simulink model "ROPOD_Control_incFlock_UDPTest"  (R2017b)
settings: Solver=ode1  StartTime=0.0  StopTime=Tfinal  FixedStep=Ts  RelTol=1e-3  EnableMultiTasking=on
PreLoadFcn:
  | init_model
InitFcn:
  | init_model
values from neighbouring files (symbols this model uses):
  AgentNumber = 1    [init_model.m]
  FFtheta_intia = 0    [init_model.m]
  FFxy_mass = 0*80    (= 0)    [init_model.m]
  I_fhz_ddelta_cntr = 0    [init_model.m]
  I_fhz_dtheta_cntr = 0.3    [init_model.m]
  I_fhz_dtheta_flock_cntr = 0.1    [init_model.m]
  I_fhz_dvarphi_cntr = 0    [init_model.m]
  I_fhz_dxdy_cntr = 0.25    [init_model.m]
  I_fhz_dxdy_flock_cntr = 0.1    [init_model.m]
  K_gain_ddelta_cntr = 0.1    [init_model.m]
  K_gain_dtheta_cntr = 150    [init_model.m]
  K_gain_dtheta_flock_cntr = 100    [init_model.m]
  K_gain_dvarphi_cntr = 0.05    [init_model.m]
  K_gain_dxdy_cntr = 200    [init_model.m]
  K_gain_dxdy_flock_cntr = 200    [init_model.m]
  LL_wp_fhz_ddelta_cntr = 2    [init_model.m]
  LL_wp_fhz_dtheta_cntr = 20    [init_model.m]
  LL_wp_fhz_dtheta_flock_cntr = 20    [init_model.m]
  LL_wp_fhz_dvarphi_cntr = 10    [init_model.m]
  LL_wp_fhz_dxdy_cntr = 20    [init_model.m]
  LL_wp_fhz_dxdy_flock_cntr = 20    [init_model.m]
  LL_wz_fhz_ddelta_cntr = 2    [init_model.m]
  LL_wz_fhz_dtheta_cntr = 20    [init_model.m]
  LL_wz_fhz_dtheta_flock_cntr = 20    [init_model.m]
  LL_wz_fhz_dvarphi_cntr = 2    [init_model.m]
  LL_wz_fhz_dxdy_cntr = 20    [init_model.m]
  LL_wz_fhz_dxdy_flock_cntr = 20    [init_model.m]
  LPF_fhz_ddelta_cntr = 50    [init_model.m]
  LPF_fhz_ddelta_meas = 50    [init_model.m]
  LPF_fhz_dtheta_cntr = 100    [init_model.m]
  LPF_fhz_dtheta_flock_cntr = 40    [init_model.m]
  LPF_fhz_dvarphi_cntr = 50    [init_model.m]
  LPF_fhz_dvarphi_meas = 50    [init_model.m]
  LPF_fhz_dxdy_cntr = 100    [init_model.m]
  LPF_fhz_dxdy_flock_cntr = 40    [init_model.m]
  max_hw_tau = 7.0    (= 7)    [init_model.m]
  max_ropod_acc_theta = 1.6    [init_model.m]
  max_ropod_acc_xy = 2.0    (= 2)    [init_model.m]
  max_ropod_sw_force = 500    [init_model.m]
  max_ropod_sw_tau = 250    [init_model.m]
  max_ropod_vel_theta = 1.6    [init_model.m]
  max_ropod_vel_xy = 2.0    (= 2)    [init_model.m]
  max_sw_current = 10    [init_model.m]
  Nagents = 2    [init_model.m]
  Nwheels = 4    [Jqwl_numeric_function.m]    (also in S_matrix.m; extract_kinmodel_parameters.m; init_model.m; tau_optimal_dist_vec_fun.m)
  pivot_offs_sws = [0.0243    0.4689    0.3384    5.9050]    [init_model.m]
  ropod_kinmodel_pv = struct2array(ropod_kinmodel_param)    [set_ropod_KinModparams.m]
  ropod_position_inflock = [-1 0 3.1416]    [init_model.m]
  SW_COM1_ENABLE1 = hex2dec('0001')    [init_model.m]
  SW_COM1_ENABLE2 = hex2dec('0002')    [init_model.m]
  SW_COM1_MODE_TORQUE = bitshift(hex2dec('0000'),2)    [init_model.m]
  SW_COM1_MODE_VELOCITY = bitshift(hex2dec('0002'),2)    [init_model.m]
  SW_COM1_USE_TS = hex2dec('8000')    [init_model.m]
  Tinit = 2    [init_model.m]
  Ts = 0.001    [init_model.m]
undefined symbols (not defined in the file or in its folder): DiscIntNeverNeededParam, sw_tau_2_curr
libraries: simulink x61, cstblocks x27, dspsigops x12, dspnetwork x4
(part 2 of 5)

== system ROPOD_Control_incFlock_UDPTest/RopodTorqueDistribution/wheel flip compensation ==
  varphi_tau_sp_in : Inport
  ropod_kin_param : Inport  Port=2
  flip_comp_factor : Inport  Port=3
  Demux : Demux  Outputs=8
  MATLAB Function : MATLAB Function  TreatAsAtomicUnit=on
  MATLAB Function1 : MATLAB Function  TreatAsAtomicUnit=on
  MATLAB Function2 : MATLAB Function  TreatAsAtomicUnit=on
  MATLAB Function3 : MATLAB Function  TreatAsAtomicUnit=on
  Mux : Mux  Inputs=8
  Terminator : Terminator
  varphi_tau_sp_out : Outport
  wires:
  varphi_tau_sp_in/1 -> Demux/1
  ropod_kin_param/1 -> [ropod_kin_param]
  flip_comp_factor/1 -> [kmax]
  Demux/2 -> MATLAB Function/2(tr)
  Demux/1 -> MATLAB Function/1(tl)
  [kmax] -> MATLAB Function/4(kmax)
  [ropod_kin_param] -> MATLAB Function/3(ropod_kinmodel_param_vec)
  Demux/4 -> MATLAB Function1/2(tr)
  Demux/3 -> MATLAB Function1/1(tl)
  [kmax] -> MATLAB Function1/4(kmax)
  [ropod_kin_param] -> MATLAB Function1/3(ropod_kinmodel_param_vec)
  Demux/6 -> MATLAB Function2/2(tr)
  Demux/5 -> MATLAB Function2/1(tl)
  [kmax] -> MATLAB Function2/4(kmax)
  [ropod_kin_param] -> MATLAB Function2/3(ropod_kinmodel_param_vec)
  Demux/8 -> MATLAB Function3/2(tr)
  Demux/7 -> MATLAB Function3/1(tl)
  [kmax] -> MATLAB Function3/4(kmax)
  [ropod_kin_param] -> MATLAB Function3/3(ropod_kinmodel_param_vec)
  MATLAB Function/1(tl_out) -> Mux/1
  MATLAB Function1/1(tl_out) -> Mux/3
  MATLAB Function2/1(tl_out) -> Mux/5
  MATLAB Function3/1(tl_out) -> Mux/7
  MATLAB Function/2(tr_out) -> Mux/2
  MATLAB Function1/2(tr_out) -> Mux/4
  MATLAB Function2/2(tr_out) -> Mux/6
  MATLAB Function3/2(tr_out) -> Mux/8
  MATLAB Function/3(sc) -> Terminator/1
  Mux/1 -> varphi_tau_sp_out/1

== system ROPOD_Control_incFlock_UDPTest/RopodVelocityController/Subscriber vel commands1 ==
  note: set 0 for testing
  note: if no vel commands are received after 0.5 sec, stop
  base_conf : Inport
  new_cmd : Inport  Port=2
  dq_setp : Inport  Port=3
  Bus Selector1 : BusSelector  OutputSignals=max_acc_xy,max_vel_xy
  Bus Selector2 : BusSelector  OutputSignals=max_acc_xy,max_vel_xy
  Bus Selector3 : BusSelector  OutputSignals=max_acc_theta,max_vel_theta
  Compare To Constant : simulink/Logic and Bit Operations/Compare To Constant  relop=>=  const=0.5  OutDataTypeStr=boolean
  Constant : Constant  Value=0  SampleTime=Ts
  Constant1 : Constant  Value=0
  Constant2 : Constant  Value=0
  Demux : Demux  Outputs=3
  Digital Clock : DigitalClock  SampleTime=Ts
  Enabled Delay : Delay  DelayLength=1  ShowEnablePort=on  SampleTime=Ts
      settings: InputPortMap=u0,e6
  Gain{,1..5} (6 alike) : Gain  Gain=-1
  Gain6 : Gain
  Mux : Mux  Inputs=3
  Rate Limiter Dynamic : simulink/Discontinuities/Rate Limiter Dynamic
      settings: SourceProductName=Simulink
  Rate Limiter Dynamic1 : simulink/Discontinuities/Rate Limiter Dynamic
      settings: SourceProductName=Simulink
  Rate Limiter Dynamic2 : simulink/Discontinuities/Rate Limiter Dynamic
      settings: SourceProductName=Simulink
  Saturation Dynamic : simulink/Discontinuities/Saturation Dynamic  OutMin=[]  OutMax=[]  OutDataTypeStr=Inherit: Same as second input  OutDataType=fixdt(1, 16)  OutScaling=2^-10  DoSatur=off
  Saturation Dynamic1 : simulink/Discontinuities/Saturation Dynamic  OutMin=[]  OutMax=[]  OutDataTypeStr=Inherit: Same as second input  OutDataType=fixdt(1, 16)  OutScaling=2^-10  DoSatur=off
  Saturation Dynamic2 : simulink/Discontinuities/Saturation Dynamic  OutMin=[]  OutMax=[]  OutDataTypeStr=Inherit: Same as second input  OutDataType=fixdt(1, 16)  OutScaling=2^-10  DoSatur=off
  Subtract : Sum  Inputs=+-
  Switch : Switch  Criteria=u2 > Threshold
  Switch1 : Switch  Criteria=u2 > Threshold
  Switch2 : Switch  Criteria=u2 > Threshold
  dq_loc : Outport
  wires:
  Demux/1 -> Switch/3
  dq_setp/1 -> Demux/1
  new_cmd/1 -> Enabled Delay/2
  Digital Clock/1 -> Enabled Delay/1, Subtract/1
  Enabled Delay/1 -> Subtract/2
  Subtract/1 -> Compare To Constant/1
  Constant/1 -> Switch/1
  Gain/1 -> Rate Limiter Dynamic/3
  Switch/1 -> Saturation Dynamic/2
  Gain1/1 -> Saturation Dynamic/3
  Saturation Dynamic/1 -> Rate Limiter Dynamic/2
  Switch1/1 -> Saturation Dynamic1/2
  Gain3/1 -> Saturation Dynamic1/3
  Constant1/1 -> Switch1/1
  Demux/2 -> Switch1/3
  Gain2/1 -> Rate Limiter Dynamic1/3
  Saturation Dynamic1/1 -> Rate Limiter Dynamic1/2
  Bus Selector2/1 -> Rate Limiter Dynamic1/1, Gain2/1  "<max_acc_xy>"
  Bus Selector2/2 -> Saturation Dynamic1/1, Gain3/1  "<max_vel_xy>"
  Bus Selector3/1 -> Rate Limiter Dynamic2/1, Gain4/1  "<max_acc_theta>"
  Saturation Dynamic2/1 -> Rate Limiter Dynamic2/2
  base_conf/1 -> Bus Selector3/1, Bus Selector2/1, Bus Selector1/1
  Switch2/1 -> Saturation Dynamic2/2
  Constant2/1 -> Switch2/1
  Demux/3 -> Switch2/3
  Gain5/1 -> Saturation Dynamic2/3
  Gain4/1 -> Rate Limiter Dynamic2/3
  Compare To Constant/1 -> Gain6/1
  Bus Selector3/2 -> Saturation Dynamic2/1, Gain5/1  "<max_vel_theta>"
  Mux/1 -> dq_loc/1
  Rate Limiter Dynamic/1 -> Mux/1
  Rate Limiter Dynamic1/1 -> Mux/2
  Rate Limiter Dynamic2/1 -> Mux/3
  Bus Selector1/2 -> Saturation Dynamic/1, Gain1/1  "<max_vel_xy>"
  Bus Selector1/1 -> Rate Limiter Dynamic/1, Gain/1  "<max_acc_xy>"
  Gain6/1 -> Switch2/2, Switch1/2, Switch/2

== system ROPOD_Control_incFlock_UDPTest/RopodVelocityController/platform vel cntr ==
  ropod_kinmodel_pv : Inport
  disable : Inport  Port=2
  platform_dxdy_cntr_param : Inport  Port=3
  platform_dtheta_cntr_param : Inport  Port=4
  platform_dxdy_cntr_param1 : Inport  Port=5
  dqr_sp : Inport  Port=6
  dqr_loc : Inport  Port=7
  delta : Inport  Port=8
  ena_w : Inport  Port=9
  dvarphi : Inport  Port=10
  Inverse Kinematics 4SW : Subsystem
  Platorm Velocity controller : Subsystem
  disable1 : InportShadow  Port=2
  wheel vel cntr : Subsystem
  w_platform_setp : Outport
  varphi_tau_setp : Outport  Port=2
  wires:
  delta/1 -> Inverse Kinematics 4SW/3(delta)
  ropod_kinmodel_pv/1 -> Inverse Kinematics 4SW/1(param_in)
  Platorm Velocity controller/1(w_platform_setp) -> w_platform_setp/1
  disable/1 -> Platorm Velocity controller/1(reset_int)
  dqr_sp/1 -> Platorm Velocity controller/2(dqr_sp), Inverse Kinematics 4SW/2(dqr_sp)
  dqr_loc/1 -> Platorm Velocity controller/3(dqr_loc)
  platform_dxdy_cntr_param/1 -> Platorm Velocity controller/4(platform_dxdy_cntr_param)
  platform_dtheta_cntr_param/1 -> Platorm Velocity controller/5(platform_dtheta_cntr_param)
  Inverse Kinematics 4SW/1(wheel_vel_sp) -> wheel vel cntr/3(dvarphi_sp)
  wheel vel cntr/1(varphi_tau_setp_out) -> varphi_tau_setp/1
  platform_dxdy_cntr_param1/1 -> wheel vel cntr/1(platform_dxdy_cntr_param)
  disable1/1 -> wheel vel cntr/2(disable)
  ena_w/1 -> wheel vel cntr/4(ena_w)
  dvarphi/1 -> wheel vel cntr/5(dvarphi)

== system ROPOD_Control_incFlock_UDPTest/Subsystem/Ropod kinematic parameters ==
  ropod_kinmodel_pv : Constant  Value=ropod_kinmodel_pv
  ropod_kin_param : Outport
  wires:
  ropod_kinmodel_pv/1 -> ropod_kin_param/1

== system ROPOD_Control_incFlock_UDPTest/Subsystem/Smart wheels conf1 ==
  Bus Creator : BusCreator  Inputs=8
  LPF_fhz_ddelta_meas : Constant  Value=LPF_fhz_ddelta_meas
  LPF_fhz_dvarphi_meas : Constant  Value=LPF_fhz_dvarphi_meas
  enable : Constant
  max_current : Constant  Value=max_sw_current
  pivot_offset_sw1 : Constant  Value=pivot_offs_sws(1)
  pivot_offset_sw2 : Constant  Value=pivot_offs_sws(2)
  pivot_offset_sw3 : Constant  Value=pivot_offs_sws(3)
  pivot_offset_sw4 : Constant  Value=pivot_offs_sws(4)
  sw_conf : Outport
  wires:
  enable/1 -> Bus Creator/1  "enable"
  Bus Creator/1 -> sw_conf/1
  max_current/1 -> Bus Creator/2  "max_current"
  pivot_offset_sw1/1 -> Bus Creator/3  "pivot_offs_sw1"
  pivot_offset_sw2/1 -> Bus Creator/4  "pivot_offs_sw2"
  pivot_offset_sw3/1 -> Bus Creator/5  "pivot_offs_sw3"
  pivot_offset_sw4/1 -> Bus Creator/6  "pivot_offs_sw4"
  LPF_fhz_dvarphi_meas/1 -> Bus Creator/7  "dvarphi_LPF_fhz"
  LPF_fhz_ddelta_meas/1 -> Bus Creator/8  "ddelta_LPF_fhz"

== system ROPOD_Control_incFlock_UDPTest/RopodTorqueDistribution/ROPOD 4SW/Initialization switch ==
  ropod_cntr_mode : Inport
  curr_setp : Inport  Port=2
  Constant1 : Constant  Value=SW_COM1_MODE_TORQUE
  Constant13 : Constant  Value=SW_COM1_MODE_TORQUE
  Constant5 : Constant  Value=SW_COM1_MODE_VELOCITY
  Index Vector : MultiPortSwitch  DataPortOrder=Zero-based contiguous  zeroidx=on
  Index Vector1 : MultiPortSwitch  DataPortOrder=Zero-based contiguous  zeroidx=on
  Movinf around SW axis center : Constant  Value=[2 -2 2 -2 2 -2 2 -2]
  zeros : Constant  Value=[0 0 0 0 0 0 0 0]
  SW_cntr_mode : Outport
  wheel_setp : Outport  Port=2
  wires:
  ropod_cntr_mode/1 -> Index Vector1/1, Index Vector/1
  Constant1/1 -> Index Vector/2
  zeros/1 -> Index Vector1/2
  Index Vector1/1 -> wheel_setp/1
  Index Vector/1 -> SW_cntr_mode/1
  Constant5/1 -> Index Vector/4
  Constant13/1 -> Index Vector/3
  Movinf around SW axis center/1 -> Index Vector1/4
  curr_setp/1 -> Index Vector1/3

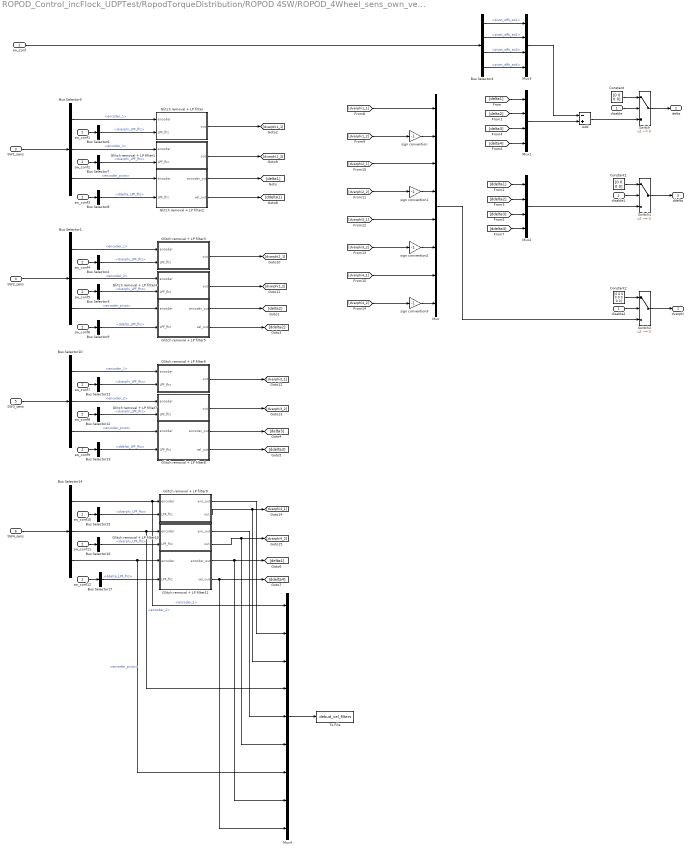
== system ROPOD_Control_incFlock_UDPTest/RopodTorqueDistribution/ROPOD 4SW/ROPOD_4Wheel_sens_own_vel_filter ==
  disable : Inport
  sw_conf : Inport  Port=2
  SW1_sens : Inport  Port=3
  SW2_sens : Inport  Port=4
  SW3_sens : Inport  Port=5
  SW4_sens : Inport  Port=6
  Add : Sum  Inputs=-+
  Bus Selector{1,5,10,14} (4 alike) : BusSelector  OutputSignals=encoder_1,encoder_2,encoder_pivot
  Bus Selector{2..3,6..7,11..12,15..16} (8 alike) : BusSelector  OutputSignals=dvarphi_LPF_fhz
  Bus Selector{8..9,13,17} (4 alike) : BusSelector  OutputSignals=ddelta_LPF_fhz
  Bus Selector4 : BusSelector  OutputSignals=pivot_offs_sw1,pivot_offs_sw2,pivot_offs_sw3,pivot_offs_sw4
  Constant : Constant  Value=[0 0 0 0]
  Constant1 : Constant  Value=[0 0 0 0]
  Constant2 : Constant  Value=[0 0 0 0 0 0 0 0]
  Glitch removal + LP filter : Subsystem
  Glitch removal + LP filter1 : Subsystem
  Glitch removal + LP filter10 : Subsystem
  Glitch removal + LP filter11 : Subsystem
  Glitch removal + LP filter2 : Subsystem
  Glitch removal + LP filter3 : Subsystem
  Glitch removal + LP filter4 : Subsystem
  Glitch removal + LP filter5 : Subsystem
  Glitch removal + LP filter6 : Subsystem
  Glitch removal + LP filter7 : Subsystem
  Glitch removal + LP filter8 : Subsystem
  Glitch removal + LP filter9 : Subsystem
  Mux : Mux  Inputs=8
  Mux1 : Mux
  Mux2 : Mux
  Mux3 : Mux
  Mux4 : Mux  Inputs=9
  Switch : Switch  Criteria=u2 ~= 0
  Switch1 : Switch  Criteria=u2 ~= 0
  Switch2 : Switch  Criteria=u2 ~= 0
  To File : ToFile  Filename=debud_vel_filters  MatrixName=debud_vel_filters
  disable1 : InportShadow
  disable2 : InportShadow
  sign convention{,1..3} (4 alike) : Gain  Gain=-1
  sw_conf{1..12} (12 alike) : InportShadow  Port=2
  dvarphi : Outport
  delta : Outport  Port=2
  ddelta : Outport  Port=3
  wires:
  SW1_sens/1 -> Bus Selector5/1
  SW2_sens/1 -> Bus Selector1/1
  [delta1] -> Mux1/1
  [delta2] -> Mux1/2
  [ddelta2] -> Mux2/2
  [ddelta1] -> Mux2/1
  SW3_sens/1 -> Bus Selector10/1
  [delta3] -> Mux1/3
  [ddelta3] -> Mux2/3
  SW4_sens/1 -> Bus Selector14/1
  [delta4] -> Mux1/4
  [ddelta4] -> Mux2/4
  Mux1/1 -> Add/2
  Mux3/1 -> Add/1
  Bus Selector4/1 -> Mux3/1  "<pivot_offs_sw1>"
  Bus Selector4/2 -> Mux3/2  "<pivot_offs_sw2>"
  Bus Selector4/3 -> Mux3/3  "<pivot_offs_sw3>"
  Bus Selector4/4 -> Mux3/4  "<pivot_offs_sw4>"
  Bus Selector5/3 -> Glitch removal + LP filter2/1(encoder)  "<encoder_pivot>"
  sign convention/1 -> Mux/2
  sign convention1/1 -> Mux/4
  sign convention2/1 -> Mux/6
  sign convention3/1 -> Mux/8
  Add/1 -> Switch/3
  Switch/1 -> delta/1
  disable/1 -> Switch/2
  Constant/1 -> Switch/1
  Switch1/1 -> ddelta/1
  Mux2/1 -> Switch1/3
  Constant1/1 -> Switch1/1
  disable1/1 -> Switch1/2
  disable2/1 -> Switch2/2
  Constant2/1 -> Switch2/1
  Mux/1 -> Switch2/3
  Switch2/1 -> dvarphi/1
  sw_conf/1 -> Bus Selector4/1
  sw_conf1/1 -> Bus Selector6/1
  sw_conf2/1 -> Bus Selector7/1
  sw_conf3/1 -> Bus Selector8/1
  sw_conf6/1 -> Bus Selector9/1
  sw_conf4/1 -> Bus Selector2/1
  sw_conf5/1 -> Bus Selector3/1
  sw_conf9/1 -> Bus Selector13/1
  sw_conf7/1 -> Bus Selector11/1
  sw_conf8/1 -> Bus Selector12/1
  sw_conf12/1 -> Bus Selector17/1
  sw_conf10/1 -> Bus Selector15/1
  sw_conf11/1 -> Bus Selector16/1
  [dvarphi1_1] -> Mux/1
  [dvarphi1_2] -> sign convention/1
  [dvarphi2_1] -> Mux/3
  [dvarphi2_2] -> sign convention1/1
  [dvarphi3_1] -> Mux/5
  [dvarphi3_2] -> sign convention2/1
  [dvarphi4_1] -> Mux/7
  [dvarphi4_2] -> sign convention3/1
  Mux4/1 -> To File/1
  Bus Selector5/1 -> Glitch removal + LP filter/1(encoder)  "<encoder_1>"
  Bus Selector6/1 -> Glitch removal + LP filter/2(LPF_fhz)  "<dvarphi_LPF_fhz>"
  Glitch removal + LP filter/1(out) -> [dvarphi1_1]
  Bus Selector7/1 -> Glitch removal + LP filter1/2(LPF_fhz)  "<dvarphi_LPF_fhz>"
  Bus Selector5/2 -> Glitch removal + LP filter1/1(encoder)  "<encoder_2>"
  Bus Selector8/1 -> Glitch removal + LP filter2/2(LPF_fhz)  "<ddelta_LPF_fhz>"
  Glitch removal + LP filter1/1(out) -> [dvarphi1_2]
  Glitch removal + LP filter2/1(encoder_out) -> [delta1]
  Glitch removal + LP filter2/2(vel_out) -> [ddelta1]
  Bus Selector2/1 -> Glitch removal + LP filter3/2(LPF_fhz)  "<dvarphi_LPF_fhz>"
  Bus Selector9/1 -> Glitch removal + LP filter5/2(LPF_fhz)  "<ddelta_LPF_fhz>"
  Bus Selector3/1 -> Glitch removal + LP filter4/2(LPF_fhz)  "<dvarphi_LPF_fhz>"
  Glitch removal + LP filter5/2(vel_out) -> [ddelta2]
  Glitch removal + LP filter3/1(out) -> [dvarphi2_1]
  Glitch removal + LP filter5/1(encoder_out) -> [delta2]
  Glitch removal + LP filter4/1(out) -> [dvarphi2_2]
  Bus Selector1/1 -> Glitch removal + LP filter3/1(encoder)  "<encoder_1>"
  Bus Selector1/2 -> Glitch removal + LP filter4/1(encoder)  "<encoder_2>"
  Bus Selector1/3 -> Glitch removal + LP filter5/1(encoder)  "<encoder_pivot>"
  Bus Selector13/1 -> Glitch removal + LP filter8/2(LPF_fhz)  "<ddelta_LPF_fhz>"
  Bus Selector10/1 -> Glitch removal + LP filter6/1(encoder)  "<encoder_1>"
  Glitch removal + LP filter7/1(out) -> [dvarphi3_2]
  Glitch removal + LP filter6/1(out) -> [dvarphi3_1]
  Bus Selector12/1 -> Glitch removal + LP filter7/2(LPF_fhz)  "<dvarphi_LPF_fhz>"
  Bus Selector10/3 -> Glitch removal + LP filter8/1(encoder)  "<encoder_pivot>"
  Glitch removal + LP filter8/1(encoder_out) -> [delta3]
  Glitch removal + LP filter8/2(vel_out) -> [ddelta3]
  Bus Selector11/1 -> Glitch removal + LP filter6/2(LPF_fhz)  "<dvarphi_LPF_fhz>"
  Bus Selector10/2 -> Glitch removal + LP filter7/1(encoder)  "<encoder_2>"
  Bus Selector17/1 -> Glitch removal + LP filter11/2(LPF_fhz)  "<ddelta_LPF_fhz>"
  Bus Selector14/1 -> Mux4/1, Glitch removal + LP filter9/1(encoder)  "<encoder_1>"
  Glitch removal + LP filter10/2(out) -> Mux4/6, [dvarphi4_2]
  Glitch removal + LP filter9/2(out) -> [dvarphi4_1], Mux4/3
  Bus Selector16/1 -> Glitch removal + LP filter10/2(LPF_fhz)  "<dvarphi_LPF_fhz>"
  Bus Selector14/3 -> Mux4/7, Glitch removal + LP filter11/1(encoder)  "<encoder_pivot>"
  Glitch removal + LP filter11/1(encoder_out) -> Mux4/8, [delta4]
  Glitch removal + LP filter11/2(vel_out) -> Mux4/9, [ddelta4]
  Bus Selector15/1 -> Glitch removal + LP filter9/2(LPF_fhz)  "<dvarphi_LPF_fhz>"
  Bus Selector14/2 -> Mux4/4, Glitch removal + LP filter10/1(encoder)  "<encoder_2>"
  Glitch removal + LP filter9/1(enc_out) -> Mux4/2
  Glitch removal + LP filter10/1(enc_out) -> Mux4/5

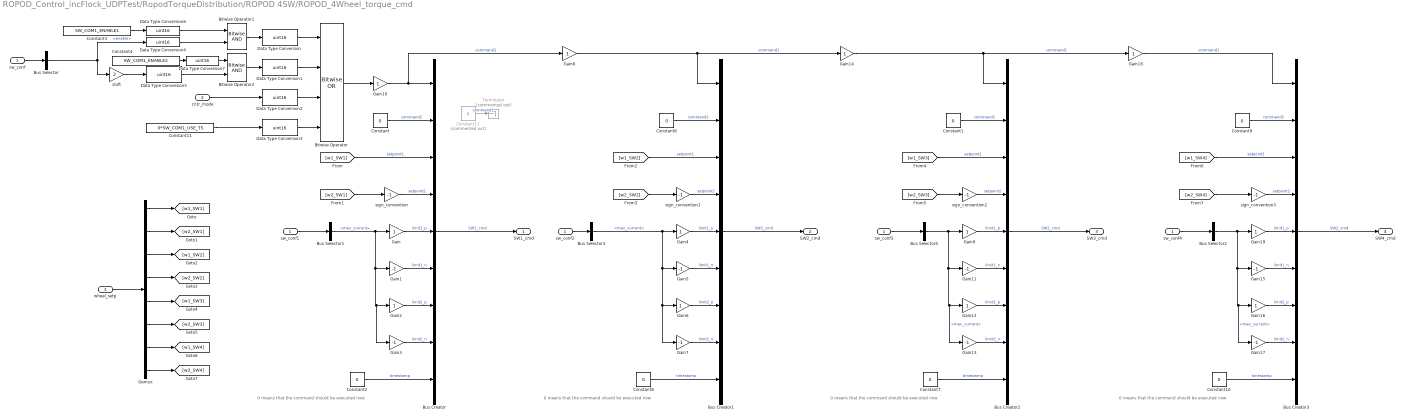
== system ROPOD_Control_incFlock_UDPTest/RopodTorqueDistribution/ROPOD 4SW/ROPOD_4Wheel_torque_cmd ==
  note: 0 means that the command should be executed now
  note: 0 means that the command should be executed now
  note: 0 means that the command should be executed now
  note: 0 means that the command should be executed now
  sw_conf : Inport
  cntr_mode : Inport  Port=2
  wheel_setp : Inport  Port=3
  Bitwise Operator : simulink/Logic and Bit Operations/Bitwise Operator  logicop=OR  UseBitMask=off  NumInputPorts=4  BitMask=bin2dec('11011001')  BitMaskRealWorld=Stored Integer
  Bitwise Operator1 : simulink/Logic and Bit Operations/Bitwise Operator  logicop=AND  UseBitMask=off  NumInputPorts=2  BitMask=bin2dec('11011001')  BitMaskRealWorld=Stored Integer
  Bitwise Operator2 : simulink/Logic and Bit Operations/Bitwise Operator  logicop=AND  UseBitMask=off  NumInputPorts=2  BitMask=bin2dec('11011001')  BitMaskRealWorld=Stored Integer
  Bus Creator{,1..3} (4 alike) : BusCreator  Inputs=9
  Bus Selector : BusSelector  OutputSignals=enable
  Bus Selector{1..4} (4 alike) : BusSelector  OutputSignals=max_current
  Constant{,1..2,6..10} (8 alike) : Constant  Value=0
  Constant11 : Constant  Value=0*SW_COM1_USE_TS
  Constant12 : Constant  Commented=on  Value=8
  Constant3 : Constant  Value=SW_COM1_ENABLE1
  Constant4 : Constant  Value=SW_COM1_ENABLE2
  Data Type Conversion{,1..7} (8 alike) : DataTypeConversion  OutDataTypeStr=uint16
  Demux : Demux  Outputs=8
  Gain{,2,4,6,9,12,16,19} (8 alike) : Gain
  Gain{1,3,5,7,11,13,15,17} (8 alike) : Gain  Gain=-1
  Gain{8,10,14,18} (4 alike) : Gain  OutDataTypeStr=double
  Terminator : Terminator  Commented=on
  shift : Gain  Gain=2
  sign_convention{,1..3} (4 alike) : Gain  Gain=-1
  sw_conf{1..4} (4 alike) : InportShadow
  SW1_cmd : Outport
  SW2_cmd : Outport  Port=2
  SW3_cmd : Outport  Port=3
  SW4_cmd : Outport  Port=4
  wires:
  Bus Creator/1 -> SW1_cmd/1  "SW1_cmd"
  Constant2/1 -> Bus Creator/9  "timestamp"
  Constant/1 -> Bus Creator/2  "command2"
  [w1_SW1] -> Bus Creator/3  "setpoint1"
  Bus Selector1/1 -> Gain3/1, Gain2/1, Gain1/1, Gain/1  "<max_current>"
  [w2_SW1] -> sign_convention/1
  [w2_SW2] -> sign_convention1/1
  [w1_SW2] -> Bus Creator1/3  "setpoint1"
  Constant6/1 -> Bus Creator1/2  "command2"
  Constant8/1 -> Bus Creator1/9  "timestamp"
  Bus Creator1/1 -> SW2_cmd/1  "SW2_cmd"
  Demux/4 -> [w2_SW2]
  Demux/1 -> [w1_SW1]
  Demux/2 -> [w2_SW1]
  Demux/3 -> [w1_SW2]
  wheel_setp/1 -> Demux/1
  Gain/1 -> Bus Creator/5  "limit1_p"
  Gain1/1 -> Bus Creator/6  "limit1_n"
  Gain2/1 -> Bus Creator/7  "limit2_p"
  Gain3/1 -> Bus Creator/8  "limit2_n"
  Gain6/1 -> Bus Creator1/7  "limit2_p"
  Gain4/1 -> Bus Creator1/5  "limit1_p"
  Gain5/1 -> Bus Creator1/6  "limit1_n"
  Gain7/1 -> Bus Creator1/8  "limit2_n"
  Bus Selector3/1 -> Gain7/1, Gain6/1, Gain5/1, Gain4/1  "<max_current>"
  Gain8/1 -> Gain14/1, Bus Creator1/1  "command1"
  Bitwise Operator/1 -> Gain10/1
  Bitwise Operator1/1 -> Data Type Conversion/1
  Data Type Conversion2/1 -> Bitwise Operator/3
  Data Type Conversion1/1 -> Bitwise Operator/2
  Data Type Conversion3/1 -> Bitwise Operator/4
  Bitwise Operator2/1 -> Data Type Conversion1/1
  Data Type Conversion/1 -> Bitwise Operator/1
  Constant11/1 -> Data Type Conversion3/1
  sw_conf/1 -> Bus Selector/1
  Bus Selector/1 -> Data Type Conversion4/1, shift/1  "<enable>"
  sw_conf1/1 -> Bus Selector1/1
  Gain10/1 -> Bus Creator/1, Gain8/1  "command1"
  sw_conf2/1 -> Bus Selector3/1
  Gain12/1 -> Bus Creator2/7  "limit2_p"
  [w2_SW3] -> sign_convention2/1
  Bus Creator2/1 -> SW3_cmd/1  "SW2_cmd"
  Gain13/1 -> Bus Creator2/8  "limit2_n"
  sw_conf3/1 -> Bus Selector4/1
  Gain11/1 -> Bus Creator2/6  "limit1_n"
  Constant1/1 -> Bus Creator2/2  "command2"
  [w1_SW3] -> Bus Creator2/3  "setpoint1"
  Constant7/1 -> Bus Creator2/9  "timestamp"
  Bus Selector4/1 -> Gain13/1, Gain12/1, Gain11/1, Gain9/1  "<max_current>"
  Gain9/1 -> Bus Creator2/5  "limit1_p"
  Demux/5 -> [w1_SW3]
  Demux/6 -> [w2_SW3]
  Gain19/1 -> Bus Creator3/5  "limit1_p"
  Bus Selector2/1 -> Gain19/1, Gain15/1, Gain16/1, Gain17/1  "<max_current>"
  Constant10/1 -> Bus Creator3/9  "timestamp"
  [w1_SW4] -> Bus Creator3/3  "setpoint1"
  Constant9/1 -> Bus Creator3/2  "command2"
  Gain15/1 -> Bus Creator3/6  "limit1_n"
  sw_conf4/1 -> Bus Selector2/1
  Gain17/1 -> Bus Creator3/8  "limit2_n"
  Bus Creator3/1 -> SW4_cmd/1  "SW2_cmd"
  [w2_SW4] -> sign_convention3/1
  Gain16/1 -> Bus Creator3/7  "limit2_p"
  Gain18/1 -> Bus Creator3/1  "command1"
  Gain14/1 -> Gain18/1, Bus Creator2/1  "command1"
  Demux/7 -> [w1_SW4]
  Demux/8 -> [w2_SW4]
  shift/1 -> Data Type Conversion5/1
  Data Type Conversion4/1 -> Bitwise Operator1/2
  Data Type Conversion5/1 -> Bitwise Operator2/2
  Constant3/1 -> Data Type Conversion6/1
  Data Type Conversion6/1 -> Bitwise Operator1/1
  Constant4/1 -> Data Type Conversion7/1
  Data Type Conversion7/1 -> Bitwise Operator2/1
  sign_convention/1 -> Bus Creator/4  "setpoint2"
  sign_convention1/1 -> Bus Creator1/4  "setpoint2"
  sign_convention2/1 -> Bus Creator2/4  "setpoint2"
  sign_convention3/1 -> Bus Creator3/4  "setpoint2"
  Constant12/1 -> Terminator/1  "command1"
  cntr_mode/1 -> Data Type Conversion2/1

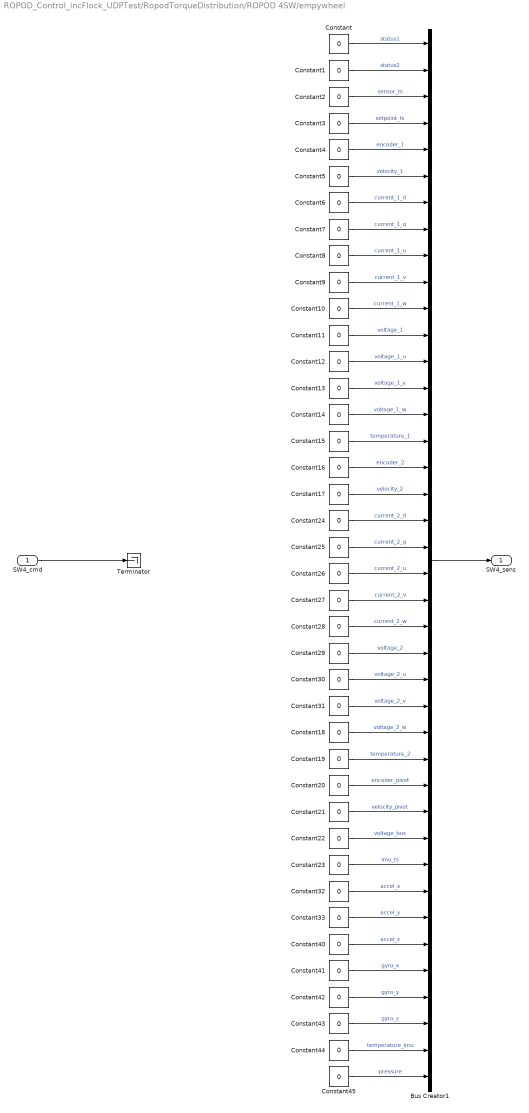
== system ROPOD_Control_incFlock_UDPTest/RopodTorqueDistribution/ROPOD 4SW/empywheel ==
  SW4_cmd : Inport
  Bus Creator1 : BusCreator  Inputs=40
  Constant{,1..33,40..45} (40 alike) : Constant  Value=0
  Terminator : Terminator
  SW4_sens : Outport
  wires:
  SW4_cmd/1 -> Terminator/1
  Constant23/1 -> Bus Creator1/32  "imu_ts"
  Constant22/1 -> Bus Creator1/31  "voltage_bus"
  Constant7/1 -> Bus Creator1/8  "current_1_q"
  Constant31/1 -> Bus Creator1/26  "voltage_2_v"
  Constant32/1 -> Bus Creator1/33  "accel_x"
  Constant15/1 -> Bus Creator1/16  "temperature_1"
  Constant44/1 -> Bus Creator1/39  "temperature_imu"
  Constant9/1 -> Bus Creator1/10  "current_1_v"
  Constant21/1 -> Bus Creator1/30  "velocity_pivot"
  Constant45/1 -> Bus Creator1/40  "pressure"
  Constant10/1 -> Bus Creator1/11  "current_1_w"
  Constant16/1 -> Bus Creator1/17  "encoder_2"
  Constant3/1 -> Bus Creator1/4  "setpoint_ts"
  Constant28/1 -> Bus Creator1/23  "current_2_w"
  Constant41/1 -> Bus Creator1/36  "gyro_x"
  Constant4/1 -> Bus Creator1/5  "encoder_1"
  Constant6/1 -> Bus Creator1/7  "current_1_d"
  Constant18/1 -> Bus Creator1/27  "voltage_2_w"
  Constant12/1 -> Bus Creator1/13  "voltage_1_u"
  Constant43/1 -> Bus Creator1/38  "gyro_z"
  Constant25/1 -> Bus Creator1/20  "current_2_q"
  Constant42/1 -> Bus Creator1/37  "gyro_y"
  Constant19/1 -> Bus Creator1/28  "temperature_2"
  Constant8/1 -> Bus Creator1/9  "current_1_u"
  Constant14/1 -> Bus Creator1/15  "voltage_1_w"
  Constant29/1 -> Bus Creator1/24  "voltage_2"
  Constant30/1 -> Bus Creator1/25  "voltage_2_u"
  Constant27/1 -> Bus Creator1/22  "current_2_v"
  Constant/1 -> Bus Creator1/1  "status1"
  Constant1/1 -> Bus Creator1/2  "status2"
  Constant40/1 -> Bus Creator1/35  "accel_z"
  Constant11/1 -> Bus Creator1/12  "voltage_1"
  Constant5/1 -> Bus Creator1/6  "velocity_1"
  Constant13/1 -> Bus Creator1/14  "voltage_1_v"
  Constant24/1 -> Bus Creator1/19  "current_2_d"
  Constant17/1 -> Bus Creator1/18  "velocity_2"
  Constant20/1 -> Bus Creator1/29  "encoder_pivot"
  Constant33/1 -> Bus Creator1/34  "accel_y"
  Constant2/1 -> Bus Creator1/3  "sensor_ts"
  Constant26/1 -> Bus Creator1/21  "current_2_u"
  Bus Creator1/1 -> SW4_sens/1

== system ROPOD_Control_incFlock_UDPTest/RopodTorqueDistribution/pivot damping cntr/Pivot controller ==
  dvarphi_error : Inport
  ena_w : Inport  Port=2
  platform_dvarphi_cntr_param : Inport  Port=3
  reset_int : Inport  Port=4
  Demux : Demux
  G_I_LL_LPF Controller1 : Subsystem
  G_I_LL_LPF Controller2 : Subsystem
  G_I_LL_LPF Controller3 : Subsystem
  G_I_LL_LPF Controller4 : Subsystem
  Gain{,6,8,10} (4 alike) : Gain  Gain=-1
  Gain{1,7,9,11} (4 alike) : Gain
  Mux : Mux  Inputs=8
  Product9 : Product
  varphi_tau_setp : Outport
  wires:
  Product9/1 -> Demux/1
  dvarphi_error/1 -> Product9/1
  [reset_int_cntr] -> G_I_LL_LPF Controller1/3(reset_integrator)
  Demux/1 -> G_I_LL_LPF Controller1/2(In)
  [param_dvarphi_cntr] -> G_I_LL_LPF Controller1/1(param)
  platform_dvarphi_cntr_param/1 -> [param_dvarphi_cntr]
  reset_int/1 -> [reset_int_cntr]
  [param_dvarphi_cntr] -> G_I_LL_LPF Controller2/1(param)
  [reset_int_cntr] -> G_I_LL_LPF Controller2/3(reset_integrator)
  Demux/2 -> G_I_LL_LPF Controller2/2(In)
  [reset_int_cntr] -> G_I_LL_LPF Controller4/3(reset_integrator)
  Demux/3 -> G_I_LL_LPF Controller3/2(In)
  Demux/4 -> G_I_LL_LPF Controller4/2(In)
  [param_dvarphi_cntr] -> G_I_LL_LPF Controller4/1(param)
  [param_dvarphi_cntr] -> G_I_LL_LPF Controller3/1(param)
  [reset_int_cntr] -> G_I_LL_LPF Controller3/3(reset_integrator)
  Mux/1 -> varphi_tau_setp/1
  ena_w/1 -> Product9/2
  G_I_LL_LPF Controller1/1(Out) -> Gain1/1, Gain/1
  G_I_LL_LPF Controller2/1(Out) -> Gain6/1, Gain7/1
  G_I_LL_LPF Controller3/1(Out) -> Gain9/1, Gain8/1
  G_I_LL_LPF Controller4/1(Out) -> Gain10/1, Gain11/1
  Gain/1 -> Mux/1
  Gain1/1 -> Mux/2
  Gain6/1 -> Mux/3
  Gain7/1 -> Mux/4
  Gain8/1 -> Mux/5
  Gain9/1 -> Mux/6
  Gain10/1 -> Mux/7
  Gain11/1 -> Mux/8

== system ROPOD_Control_incFlock_UDPTest/RopodVelocityController/platform vel cntr/Inverse Kinematics 4SW ==
  param_in : Inport
  dqr_sp : Inport  Port=2
  delta : Inport  Port=3
  Gl_matrix : MATLAB Function  TreatAsAtomicUnit=on
  Product3 : Product  Multiplication=Matrix(*)
  Selector2 : Selector  IndexMode=Zero-based  InputPortWidth=3+3*Nwheels  IndexOptions=Index vector (dialog)  Indices=[3+Nwheels:3+3*Nwheels-1]  OutputSizes=1
  wheel_vel_sp : Outport
  wires:
  param_in/1 -> Gl_matrix/1(ropod_kinmodel_param_vec)
  Gl_matrix/1(Gl) -> Product3/1
  Product3/1 -> Selector2/1
  delta/1 -> Gl_matrix/2(delta)
  dqr_sp/1 -> Product3/2
  Selector2/1 -> wheel_vel_sp/1

== system ROPOD_Control_incFlock_UDPTest/RopodVelocityController/platform vel cntr/Platorm Velocity controller ==
  note: Mass Feedforward
  reset_int : Inport
  dqr_sp : Inport  Port=2
  dqr_loc : Inport  Port=3
  platform_dxdy_cntr_param : Inport  Port=4
  platform_dtheta_cntr_param : Inport  Port=5
  Demux : Demux  Outputs=3
  Demux1 : Demux  Outputs=3
  Discrete Derivative : simulink/Discrete/Discrete Derivative  gainval=1.0  ICPrevScaledInput=0.0  OutMin=[]  OutMax=[]  OutDataType=fixdt(1, 16)  OutScaling=2^-10  DoSatur=off
  G_I_LL_LPF Controller_X : Subsystem
  G_I_LL_LPF Controller_Y : Subsystem
  G_I_LL_LPF Controller_theta : Subsystem
  Gain : Gain  Gain=FFxy_mass
  Gain1 : Gain  Gain=FFxy_mass
  Gain2 : Gain  Gain=FFtheta_intia
  Mux : Mux  Inputs=3
  Mux1 : Mux  Inputs=3
  Sum : Sum  Inputs=|+-
  Sum1 : Sum  Inputs=++|
  w_platform_setp : Outport
  wires:
  Sum/1 -> Demux/1
  G_I_LL_LPF Controller_theta/1(Out) -> Mux/3
  Demux/1 -> G_I_LL_LPF Controller_X/2(In)
  Demux/2 -> G_I_LL_LPF Controller_Y/2(In)
  G_I_LL_LPF Controller_Y/1(Out) -> Mux/2
  G_I_LL_LPF Controller_X/1(Out) -> Mux/1
  Demux/3 -> G_I_LL_LPF Controller_theta/2(In)
  dqr_sp/1 -> Sum/1, Discrete Derivative/1
  dqr_loc/1 -> Sum/2
  [param_dxdy_cntr] -> G_I_LL_LPF Controller_X/1(param)
  [param_dxdy_cntr] -> G_I_LL_LPF Controller_Y/1(param)
  [param_dtheta_cntr] -> G_I_LL_LPF Controller_theta/1(param)
  reset_int/1 -> [reset_int_cntr]
  [reset_int_cntr] -> G_I_LL_LPF Controller_X/3(reset_integrator)
  [reset_int_cntr] -> G_I_LL_LPF Controller_Y/3(reset_integrator)
  platform_dxdy_cntr_param/1 -> [param_dxdy_cntr]
  platform_dtheta_cntr_param/1 -> [param_dtheta_cntr]
  [reset_int_cntr] -> G_I_LL_LPF Controller_theta/3(reset_integrator)
  Discrete Derivative/1 -> Demux1/1
  Demux1/1 -> Gain/1
  Gain/1 -> Mux1/1
  Demux1/2 -> Gain1/1
  Gain1/1 -> Mux1/2
  Demux1/3 -> Gain2/1
  Gain2/1 -> Mux1/3
  Sum1/1 -> w_platform_setp/1
  Mux1/1 -> Sum1/1
  Mux/1 -> Sum1/2

== system ROPOD_Control_incFlock_UDPTest/RopodVelocityController/platform vel cntr/wheel vel cntr ==
  platform_dxdy_cntr_param : Inport
  disable : Inport  Port=2
  dvarphi_sp : Inport  Port=3
  ena_w : Inport  Port=4
  dvarphi : Inport  Port=5
  Sum : Sum  Inputs=-+|
  Wheels Velocity controller : Subsystem
  varphi_tau_setp_out : Outport
  wires:
  Wheels Velocity controller/1(varphi_tau_setp) -> varphi_tau_setp_out/1
  ena_w/1 -> Wheels Velocity controller/2(ena_w)
  Sum/1 -> Wheels Velocity controller/1(dvarphi_error)
  dvarphi/1 -> Sum/1
  dvarphi_sp/1 -> Sum/2
  disable/1 -> Wheels Velocity controller/4(reset_int)
  platform_dxdy_cntr_param/1 -> Wheels Velocity controller/3(platform_dvarphi_cntr_param)

== system ROPOD_Control_incFlock_UDPTest/RopodTorqueDistribution/ROPOD 4SW/ROPOD_4Wheel_sens_own_vel_filter/Glitch removal + LP filter ==
  encoder : Inport
  LPF_fhz : Inport  Port=2
  Constant3 : Constant  Value=Ts
  Discrete Derivative : simulink/Discrete/Discrete Derivative  gainval=1  ICPrevScaledInput=0.0  OutMin=[]  OutMax=[]  OutDataType=fixdt(1, 16)  OutScaling=2^-10  DoSatur=off
  Discrete Varying Lowpass12 : cstblocks/Linear Parameter Varying/Discrete Varying Lowpass  N=2  w0=0  Ts=Ts
      settings: SourceProductName=Control System Toolbox  SourceProductBaseCode=CT
  Remove_glitches1 : MATLAB Function  TreatAsAtomicUnit=on
  Unit Delay : UnitDelay  SampleTime=-1
  Unwrap11 : dspsigops/Unwrap  tol=0.1  running=on
  sign convention4 : Gain  Gain=2*pi
  out : Outport
  wires:
  Unit Delay/1 -> Remove_glitches1/1(vel)
  sign convention4/1 -> Discrete Varying Lowpass12/2
  Unwrap11/1 -> Remove_glitches1/3(encoder)
  LPF_fhz/1 -> sign convention4/1
  Remove_glitches1/1(encoder_out) -> Discrete Derivative/1
  Constant3/1 -> Remove_glitches1/2(Ts)
  Discrete Varying Lowpass12/1 -> out/1
  encoder/1 -> Unwrap11/1
  Discrete Derivative/1 -> Unit Delay/1, Discrete Varying Lowpass12/1

== system ROPOD_Control_incFlock_UDPTest/RopodTorqueDistribution/ROPOD 4SW/ROPOD_4Wheel_sens_own_vel_filter/Glitch removal + LP filter1 ==
  encoder : Inport
  LPF_fhz : Inport  Port=2
  Constant3 : Constant  Value=Ts
  Discrete Derivative : simulink/Discrete/Discrete Derivative  gainval=1  ICPrevScaledInput=0.0  OutMin=[]  OutMax=[]  OutDataType=fixdt(1, 16)  OutScaling=2^-10  DoSatur=off
  Discrete Varying Lowpass12 : cstblocks/Linear Parameter Varying/Discrete Varying Lowpass  N=2  w0=0  Ts=Ts
      settings: SourceProductName=Control System Toolbox  SourceProductBaseCode=CT
  Remove_glitches1 : MATLAB Function  TreatAsAtomicUnit=on
  Unit Delay : UnitDelay  SampleTime=-1
  Unwrap11 : dspsigops/Unwrap  tol=0.1  running=on
  sign convention4 : Gain  Gain=2*pi
  out : Outport
  wires:
  Discrete Derivative/1 -> Discrete Varying Lowpass12/1, Unit Delay/1
  encoder/1 -> Unwrap11/1
  Discrete Varying Lowpass12/1 -> out/1
  Constant3/1 -> Remove_glitches1/2(Ts)
  Remove_glitches1/1(encoder_out) -> Discrete Derivative/1
  LPF_fhz/1 -> sign convention4/1
  Unwrap11/1 -> Remove_glitches1/3(encoder)
  sign convention4/1 -> Discrete Varying Lowpass12/2
  Unit Delay/1 -> Remove_glitches1/1(vel)

== system ROPOD_Control_incFlock_UDPTest/RopodTorqueDistribution/ROPOD 4SW/ROPOD_4Wheel_sens_own_vel_filter/Glitch removal + LP filter10 ==
  encoder : Inport
  LPF_fhz : Inport  Port=2
  Constant3 : Constant  Value=Ts
  Discrete Derivative : simulink/Discrete/Discrete Derivative  gainval=1  ICPrevScaledInput=0.0  OutMin=[]  OutMax=[]  OutDataType=fixdt(1, 16)  OutScaling=2^-10  DoSatur=off
  Discrete Varying Lowpass12 : cstblocks/Linear Parameter Varying/Discrete Varying Lowpass  N=2  w0=0  Ts=Ts
      settings: SourceProductName=Control System Toolbox  SourceProductBaseCode=CT
  Remove_glitches1 : MATLAB Function  TreatAsAtomicUnit=on
  Unit Delay : UnitDelay  SampleTime=-1
  Unwrap11 : dspsigops/Unwrap  tol=0.1  running=on
  sign convention4 : Gain  Gain=2*pi
  enc_out : Outport
  out : Outport  Port=2
  wires:
  Unit Delay/1 -> Remove_glitches1/1(vel)
  sign convention4/1 -> Discrete Varying Lowpass12/2
  Unwrap11/1 -> Remove_glitches1/3(encoder)
  LPF_fhz/1 -> sign convention4/1
  Remove_glitches1/1(encoder_out) -> enc_out/1, Discrete Derivative/1
  Constant3/1 -> Remove_glitches1/2(Ts)
  Discrete Varying Lowpass12/1 -> out/1
  encoder/1 -> Unwrap11/1
  Discrete Derivative/1 -> Unit Delay/1, Discrete Varying Lowpass12/1

== system ROPOD_Control_incFlock_UDPTest/RopodTorqueDistribution/ROPOD 4SW/ROPOD_4Wheel_sens_own_vel_filter/Glitch removal + LP filter11 ==
  encoder : Inport
  LPF_fhz : Inport  Port=2
  Constant3 : Constant  Value=Ts
  Discrete Derivative : simulink/Discrete/Discrete Derivative  gainval=1  ICPrevScaledInput=0.0  OutMin=[]  OutMax=[]  OutDataType=fixdt(1, 16)  OutScaling=2^-10  DoSatur=off
  Discrete Varying Lowpass12 : cstblocks/Linear Parameter Varying/Discrete Varying Lowpass  N=2  w0=0  Ts=Ts
      settings: SourceProductName=Control System Toolbox  SourceProductBaseCode=CT
  Remove_glitches1 : MATLAB Function  TreatAsAtomicUnit=on
  Unit Delay : UnitDelay  SampleTime=-1
  Unwrap11 : dspsigops/Unwrap  tol=0.1  running=on
  sign convention4 : Gain  Gain=2*pi
  encoder_out : Outport
  vel_out : Outport  Port=2
  wires:
  Unit Delay/1 -> Remove_glitches1/1(vel)
  sign convention4/1 -> Discrete Varying Lowpass12/2
  Unwrap11/1 -> Remove_glitches1/3(encoder)
  LPF_fhz/1 -> sign convention4/1
  Remove_glitches1/1(encoder_out) -> encoder_out/1, Discrete Derivative/1
  Constant3/1 -> Remove_glitches1/2(Ts)
  Discrete Varying Lowpass12/1 -> vel_out/1
  encoder/1 -> Unwrap11/1
  Discrete Derivative/1 -> Unit Delay/1, Discrete Varying Lowpass12/1

== system ROPOD_Control_incFlock_UDPTest/RopodTorqueDistribution/ROPOD 4SW/ROPOD_4Wheel_sens_own_vel_filter/Glitch removal + LP filter2 ==
  encoder : Inport
  LPF_fhz : Inport  Port=2
  Constant3 : Constant  Value=Ts
  Discrete Derivative : simulink/Discrete/Discrete Derivative  gainval=1  ICPrevScaledInput=0.0  OutMin=[]  OutMax=[]  OutDataType=fixdt(1, 16)  OutScaling=2^-10  DoSatur=off
  Discrete Varying Lowpass12 : cstblocks/Linear Parameter Varying/Discrete Varying Lowpass  N=2  w0=0  Ts=Ts
      settings: SourceProductName=Control System Toolbox  SourceProductBaseCode=CT
  Remove_glitches1 : MATLAB Function  TreatAsAtomicUnit=on
  Unit Delay : UnitDelay  SampleTime=-1
  Unwrap11 : dspsigops/Unwrap  tol=0.1  running=on
  sign convention4 : Gain  Gain=2*pi
  encoder_out : Outport
  vel_out : Outport  Port=2
  wires:
  Unit Delay/1 -> Remove_glitches1/1(vel)
  sign convention4/1 -> Discrete Varying Lowpass12/2
  Unwrap11/1 -> Remove_glitches1/3(encoder)
  LPF_fhz/1 -> sign convention4/1
  Remove_glitches1/1(encoder_out) -> encoder_out/1, Discrete Derivative/1
  Constant3/1 -> Remove_glitches1/2(Ts)
  Discrete Varying Lowpass12/1 -> vel_out/1
  encoder/1 -> Unwrap11/1
  Discrete Derivative/1 -> Unit Delay/1, Discrete Varying Lowpass12/1

== system ROPOD_Control_incFlock_UDPTest/RopodTorqueDistribution/ROPOD 4SW/ROPOD_4Wheel_sens_own_vel_filter/Glitch removal + LP filter3 ==
  encoder : Inport
  LPF_fhz : Inport  Port=2
  Constant3 : Constant  Value=Ts
  Discrete Derivative : simulink/Discrete/Discrete Derivative  gainval=1  ICPrevScaledInput=0.0  OutMin=[]  OutMax=[]  OutDataType=fixdt(1, 16)  OutScaling=2^-10  DoSatur=off
  Discrete Varying Lowpass12 : cstblocks/Linear Parameter Varying/Discrete Varying Lowpass  N=2  w0=0  Ts=Ts
      settings: SourceProductName=Control System Toolbox  SourceProductBaseCode=CT
  Remove_glitches1 : MATLAB Function  TreatAsAtomicUnit=on
  Unit Delay : UnitDelay  SampleTime=-1
  Unwrap11 : dspsigops/Unwrap  tol=0.1  running=on
  sign convention4 : Gain  Gain=2*pi
  out : Outport
  wires:
  Unit Delay/1 -> Remove_glitches1/1(vel)
  sign convention4/1 -> Discrete Varying Lowpass12/2
  Unwrap11/1 -> Remove_glitches1/3(encoder)
  LPF_fhz/1 -> sign convention4/1
  Remove_glitches1/1(encoder_out) -> Discrete Derivative/1
  Constant3/1 -> Remove_glitches1/2(Ts)
  Discrete Varying Lowpass12/1 -> out/1
  encoder/1 -> Unwrap11/1
  Discrete Derivative/1 -> Unit Delay/1, Discrete Varying Lowpass12/1

== system ROPOD_Control_incFlock_UDPTest/RopodTorqueDistribution/ROPOD 4SW/ROPOD_4Wheel_sens_own_vel_filter/Glitch removal + LP filter4 ==
  encoder : Inport
  LPF_fhz : Inport  Port=2
  Constant3 : Constant  Value=Ts
  Discrete Derivative : simulink/Discrete/Discrete Derivative  gainval=1  ICPrevScaledInput=0.0  OutMin=[]  OutMax=[]  OutDataType=fixdt(1, 16)  OutScaling=2^-10  DoSatur=off
  Discrete Varying Lowpass12 : cstblocks/Linear Parameter Varying/Discrete Varying Lowpass  N=2  w0=0  Ts=Ts
      settings: SourceProductName=Control System Toolbox  SourceProductBaseCode=CT
  Remove_glitches1 : MATLAB Function  TreatAsAtomicUnit=on
  Unit Delay : UnitDelay  SampleTime=-1
  Unwrap11 : dspsigops/Unwrap  tol=0.1  running=on
  sign convention4 : Gain  Gain=2*pi
  out : Outport
  wires:
  Discrete Derivative/1 -> Discrete Varying Lowpass12/1, Unit Delay/1
  encoder/1 -> Unwrap11/1
  Discrete Varying Lowpass12/1 -> out/1
  Constant3/1 -> Remove_glitches1/2(Ts)
  Remove_glitches1/1(encoder_out) -> Discrete Derivative/1
  LPF_fhz/1 -> sign convention4/1
  Unwrap11/1 -> Remove_glitches1/3(encoder)
  sign convention4/1 -> Discrete Varying Lowpass12/2
  Unit Delay/1 -> Remove_glitches1/1(vel)

== system ROPOD_Control_incFlock_UDPTest/RopodTorqueDistribution/ROPOD 4SW/ROPOD_4Wheel_sens_own_vel_filter/Glitch removal + LP filter5 ==
  encoder : Inport
  LPF_fhz : Inport  Port=2
  Constant3 : Constant  Value=Ts
  Discrete Derivative : simulink/Discrete/Discrete Derivative  gainval=1  ICPrevScaledInput=0.0  OutMin=[]  OutMax=[]  OutDataType=fixdt(1, 16)  OutScaling=2^-10  DoSatur=off
  Discrete Varying Lowpass12 : cstblocks/Linear Parameter Varying/Discrete Varying Lowpass  N=2  w0=0  Ts=Ts
      settings: SourceProductName=Control System Toolbox  SourceProductBaseCode=CT
  Remove_glitches1 : MATLAB Function  TreatAsAtomicUnit=on
  Unit Delay : UnitDelay  SampleTime=-1
  Unwrap11 : dspsigops/Unwrap  tol=0.1  running=on
  sign convention4 : Gain  Gain=2*pi
  encoder_out : Outport
  vel_out : Outport  Port=2
  wires:
  Unit Delay/1 -> Remove_glitches1/1(vel)
  sign convention4/1 -> Discrete Varying Lowpass12/2
  Unwrap11/1 -> Remove_glitches1/3(encoder)
  LPF_fhz/1 -> sign convention4/1
  Remove_glitches1/1(encoder_out) -> encoder_out/1, Discrete Derivative/1
  Constant3/1 -> Remove_glitches1/2(Ts)
  Discrete Varying Lowpass12/1 -> vel_out/1
  encoder/1 -> Unwrap11/1
  Discrete Derivative/1 -> Unit Delay/1, Discrete Varying Lowpass12/1

== system ROPOD_Control_incFlock_UDPTest/RopodTorqueDistribution/ROPOD 4SW/ROPOD_4Wheel_sens_own_vel_filter/Glitch removal + LP filter6 ==
  encoder : Inport
  LPF_fhz : Inport  Port=2
  Constant3 : Constant  Value=Ts
  Discrete Derivative : simulink/Discrete/Discrete Derivative  gainval=1  ICPrevScaledInput=0.0  OutMin=[]  OutMax=[]  OutDataType=fixdt(1, 16)  OutScaling=2^-10  DoSatur=off
  Discrete Varying Lowpass12 : cstblocks/Linear Parameter Varying/Discrete Varying Lowpass  N=2  w0=0  Ts=Ts
      settings: SourceProductName=Control System Toolbox  SourceProductBaseCode=CT
  Remove_glitches1 : MATLAB Function  TreatAsAtomicUnit=on
  Unit Delay : UnitDelay  SampleTime=-1
  Unwrap11 : dspsigops/Unwrap  tol=0.1  running=on
  sign convention4 : Gain  Gain=2*pi
  out : Outport
  wires:
  Unit Delay/1 -> Remove_glitches1/1(vel)
  sign convention4/1 -> Discrete Varying Lowpass12/2
  Unwrap11/1 -> Remove_glitches1/3(encoder)
  LPF_fhz/1 -> sign convention4/1
  Remove_glitches1/1(encoder_out) -> Discrete Derivative/1
  Constant3/1 -> Remove_glitches1/2(Ts)
  Discrete Varying Lowpass12/1 -> out/1
  encoder/1 -> Unwrap11/1
  Discrete Derivative/1 -> Unit Delay/1, Discrete Varying Lowpass12/1

== system ROPOD_Control_incFlock_UDPTest/RopodTorqueDistribution/ROPOD 4SW/ROPOD_4Wheel_sens_own_vel_filter/Glitch removal + LP filter7 ==
  encoder : Inport
  LPF_fhz : Inport  Port=2
  Constant3 : Constant  Value=Ts
  Discrete Derivative : simulink/Discrete/Discrete Derivative  gainval=1  ICPrevScaledInput=0.0  OutMin=[]  OutMax=[]  OutDataType=fixdt(1, 16)  OutScaling=2^-10  DoSatur=off
  Discrete Varying Lowpass12 : cstblocks/Linear Parameter Varying/Discrete Varying Lowpass  N=2  w0=0  Ts=Ts
      settings: SourceProductName=Control System Toolbox  SourceProductBaseCode=CT
  Remove_glitches1 : MATLAB Function  TreatAsAtomicUnit=on
  Unit Delay : UnitDelay  SampleTime=-1
  Unwrap11 : dspsigops/Unwrap  tol=0.1  running=on
  sign convention4 : Gain  Gain=2*pi
  out : Outport
  wires:
  Discrete Derivative/1 -> Discrete Varying Lowpass12/1, Unit Delay/1
  encoder/1 -> Unwrap11/1
  Discrete Varying Lowpass12/1 -> out/1
  Constant3/1 -> Remove_glitches1/2(Ts)
  Remove_glitches1/1(encoder_out) -> Discrete Derivative/1
  LPF_fhz/1 -> sign convention4/1
  Unwrap11/1 -> Remove_glitches1/3(encoder)
  sign convention4/1 -> Discrete Varying Lowpass12/2
  Unit Delay/1 -> Remove_glitches1/1(vel)

== system ROPOD_Control_incFlock_UDPTest/RopodTorqueDistribution/ROPOD 4SW/ROPOD_4Wheel_sens_own_vel_filter/Glitch removal + LP filter8 ==
  encoder : Inport
  LPF_fhz : Inport  Port=2
  Constant3 : Constant  Value=Ts
  Discrete Derivative : simulink/Discrete/Discrete Derivative  gainval=1  ICPrevScaledInput=0.0  OutMin=[]  OutMax=[]  OutDataType=fixdt(1, 16)  OutScaling=2^-10  DoSatur=off
  Discrete Varying Lowpass12 : cstblocks/Linear Parameter Varying/Discrete Varying Lowpass  N=2  w0=0  Ts=Ts
      settings: SourceProductName=Control System Toolbox  SourceProductBaseCode=CT
  Remove_glitches1 : MATLAB Function  TreatAsAtomicUnit=on
  Unit Delay : UnitDelay  SampleTime=-1
  Unwrap11 : dspsigops/Unwrap  tol=0.1  running=on
  sign convention4 : Gain  Gain=2*pi
  encoder_out : Outport
  vel_out : Outport  Port=2
  wires:
  Unit Delay/1 -> Remove_glitches1/1(vel)
  sign convention4/1 -> Discrete Varying Lowpass12/2
  Unwrap11/1 -> Remove_glitches1/3(encoder)
  LPF_fhz/1 -> sign convention4/1
  Remove_glitches1/1(encoder_out) -> encoder_out/1, Discrete Derivative/1
  Constant3/1 -> Remove_glitches1/2(Ts)
  Discrete Varying Lowpass12/1 -> vel_out/1
  encoder/1 -> Unwrap11/1
  Discrete Derivative/1 -> Unit Delay/1, Discrete Varying Lowpass12/1

== system ROPOD_Control_incFlock_UDPTest/RopodTorqueDistribution/ROPOD 4SW/ROPOD_4Wheel_sens_own_vel_filter/Glitch removal + LP filter9 ==
  encoder : Inport
  LPF_fhz : Inport  Port=2
  Constant3 : Constant  Value=Ts
  Discrete Derivative : simulink/Discrete/Discrete Derivative  gainval=1  ICPrevScaledInput=0.0  OutMin=[]  OutMax=[]  OutDataType=fixdt(1, 16)  OutScaling=2^-10  DoSatur=off
  Discrete Varying Lowpass12 : cstblocks/Linear Parameter Varying/Discrete Varying Lowpass  N=2  w0=0  Ts=Ts
      settings: SourceProductName=Control System Toolbox  SourceProductBaseCode=CT
  Remove_glitches1 : MATLAB Function  TreatAsAtomicUnit=on
  Unit Delay : UnitDelay  SampleTime=-1
  Unwrap11 : dspsigops/Unwrap  tol=0.1  running=on
  sign convention4 : Gain  Gain=2*pi
  enc_out : Outport
  out : Outport  Port=2
  wires:
  Unit Delay/1 -> Remove_glitches1/1(vel)
  sign convention4/1 -> Discrete Varying Lowpass12/2
  Unwrap11/1 -> Remove_glitches1/3(encoder)
  LPF_fhz/1 -> sign convention4/1
  Remove_glitches1/1(encoder_out) -> enc_out/1, Discrete Derivative/1
  Constant3/1 -> Remove_glitches1/2(Ts)
  Discrete Varying Lowpass12/1 -> out/1
  encoder/1 -> Unwrap11/1
  Discrete Derivative/1 -> Unit Delay/1, Discrete Varying Lowpass12/1

== system ROPOD_Control_incFlock_UDPTest/RopodTorqueDistribution/pivot damping cntr/Pivot controller/G_I_LL_LPF Controller1 ==
  param : Inport
  In : Inport  Port=2
  reset_integrator : Inport  Port=3
  Bus Selector : BusSelector  OutputSignals=P_gain,I_freq_hz,LL_zero_fhz,LL_pole_fhz,LPF_fhz
  Discrete Varying Lowpass3 : cstblocks/Linear Parameter Varying/Discrete Varying Lowpass  N=1  w0=0  Ts=Ts
      settings: SourceProductName=Control System Toolbox  SourceProductBaseCode=CT
  Gain2 : Gain  Gain=2*pi
  Product5 : Product
  Shapeit Integrator (Tustin) : Subsystem
  Shapeit Lead-Lag (Tustin) : Subsystem
  Out : Outport
  wires:
  Gain2/1 -> Discrete Varying Lowpass3/2
  Product5/1 -> Shapeit Integrator (Tustin)/1(In)
  Discrete Varying Lowpass3/1 -> Out/1
  Shapeit Integrator (Tustin)/1(Out) -> Shapeit Lead-Lag (Tustin)/1(In)
  Bus Selector/1 -> Product5/2  "<P_gain>"
  Bus Selector/2 -> Shapeit Integrator (Tustin)/2(I_fhz)  "<I_freq_hz>"
  param/1 -> Bus Selector/1
  Bus Selector/5 -> Gain2/1  "<LPF_fhz>"
  Bus Selector/4 -> Shapeit Lead-Lag (Tustin)/3(fp)  "<LL_pole_fhz>"
  reset_integrator/1 -> Shapeit Integrator (Tustin)/3(reset)
  Bus Selector/3 -> Shapeit Lead-Lag (Tustin)/2(fz)  "<LL_zero_fhz>"
  Shapeit Lead-Lag (Tustin)/1(Out) -> Discrete Varying Lowpass3/1
  In/1 -> Product5/1

== system ROPOD_Control_incFlock_UDPTest/RopodTorqueDistribution/pivot damping cntr/Pivot controller/G_I_LL_LPF Controller2 ==
  param : Inport
  In : Inport  Port=2
  reset_integrator : Inport  Port=3
  Bus Selector : BusSelector  OutputSignals=P_gain,I_freq_hz,LL_zero_fhz,LL_pole_fhz,LPF_fhz
  Discrete Varying Lowpass3 : cstblocks/Linear Parameter Varying/Discrete Varying Lowpass  N=1  w0=0  Ts=Ts
      settings: SourceProductName=Control System Toolbox  SourceProductBaseCode=CT
  Gain2 : Gain  Gain=2*pi
  Product5 : Product
  Shapeit Integrator (Tustin) : Subsystem
  Shapeit Lead-Lag (Tustin) : Subsystem
  Out : Outport
  wires:
  Gain2/1 -> Discrete Varying Lowpass3/2
  Product5/1 -> Shapeit Integrator (Tustin)/1(In)
  Discrete Varying Lowpass3/1 -> Out/1
  Shapeit Integrator (Tustin)/1(Out) -> Shapeit Lead-Lag (Tustin)/1(In)
  Bus Selector/1 -> Product5/2  "<P_gain>"
  Bus Selector/2 -> Shapeit Integrator (Tustin)/2(I_fhz)  "<I_freq_hz>"
  param/1 -> Bus Selector/1
  Bus Selector/5 -> Gain2/1  "<LPF_fhz>"
  Bus Selector/4 -> Shapeit Lead-Lag (Tustin)/3(fp)  "<LL_pole_fhz>"
  reset_integrator/1 -> Shapeit Integrator (Tustin)/3(reset)
  Bus Selector/3 -> Shapeit Lead-Lag (Tustin)/2(fz)  "<LL_zero_fhz>"
  Shapeit Lead-Lag (Tustin)/1(Out) -> Discrete Varying Lowpass3/1
  In/1 -> Product5/1

== system ROPOD_Control_incFlock_UDPTest/RopodTorqueDistribution/pivot damping cntr/Pivot controller/G_I_LL_LPF Controller3 ==
  param : Inport
  In : Inport  Port=2
  reset_integrator : Inport  Port=3
  Bus Selector : BusSelector  OutputSignals=P_gain,I_freq_hz,LL_zero_fhz,LL_pole_fhz,LPF_fhz
  Discrete Varying Lowpass3 : cstblocks/Linear Parameter Varying/Discrete Varying Lowpass  N=1  w0=0  Ts=Ts
      settings: SourceProductName=Control System Toolbox  SourceProductBaseCode=CT
  Gain2 : Gain  Gain=2*pi
  Product5 : Product
  Shapeit Integrator (Tustin) : Subsystem
  Shapeit Lead-Lag (Tustin) : Subsystem
  Out : Outport
  wires:
  In/1 -> Product5/1
  Shapeit Lead-Lag (Tustin)/1(Out) -> Discrete Varying Lowpass3/1
  Bus Selector/3 -> Shapeit Lead-Lag (Tustin)/2(fz)  "<LL_zero_fhz>"
  reset_integrator/1 -> Shapeit Integrator (Tustin)/3(reset)
  Bus Selector/4 -> Shapeit Lead-Lag (Tustin)/3(fp)  "<LL_pole_fhz>"
  Bus Selector/5 -> Gain2/1  "<LPF_fhz>"
  param/1 -> Bus Selector/1
  Bus Selector/2 -> Shapeit Integrator (Tustin)/2(I_fhz)  "<I_freq_hz>"
  Bus Selector/1 -> Product5/2  "<P_gain>"
  Shapeit Integrator (Tustin)/1(Out) -> Shapeit Lead-Lag (Tustin)/1(In)
  Discrete Varying Lowpass3/1 -> Out/1
  Product5/1 -> Shapeit Integrator (Tustin)/1(In)
  Gain2/1 -> Discrete Varying Lowpass3/2
